simulink model "simulator_quarternions"  (R2025b)
settings: Solver=FixedStepAuto  StartTime=0.0  StopTime=15  FixedStep=0.01  RelTol=1e-3
values from neighbouring files (symbols this model uses):
  omega0 = qdot0    [model_init.m]
  q0_quat = euler2quat(q0)    [model_init.m]
  u0 = system_params.u0(i)    [Q_tension_calc.m]    (also in Tau_tension_calc.m; model_init.m = u0_calc(q0, system_params); u0_calc.m = zeros(size(fields)))
  u_offset = [106; 80; 79; 75; 67; 72; 80]/1000 - u0_calc(q_neutral, system_params)    [model_init.m]
undefined symbols (not defined in the file or in its folder): Cd, Dd, EKF_settings, Jm, Ke, Km, Mf, Ml, P0, Ra, system_params, u0_mpc, x0_EKF
libraries: mpclib x1
settings Model: Creator=Sigbjørn  LastModifiedBy=sig

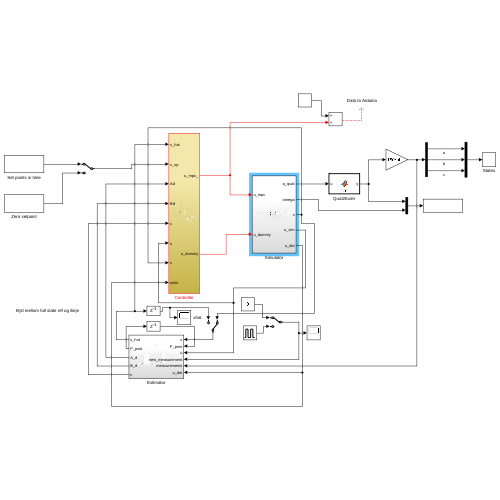
[thumbnail: Simulink's stored preview of the top-level diagram]
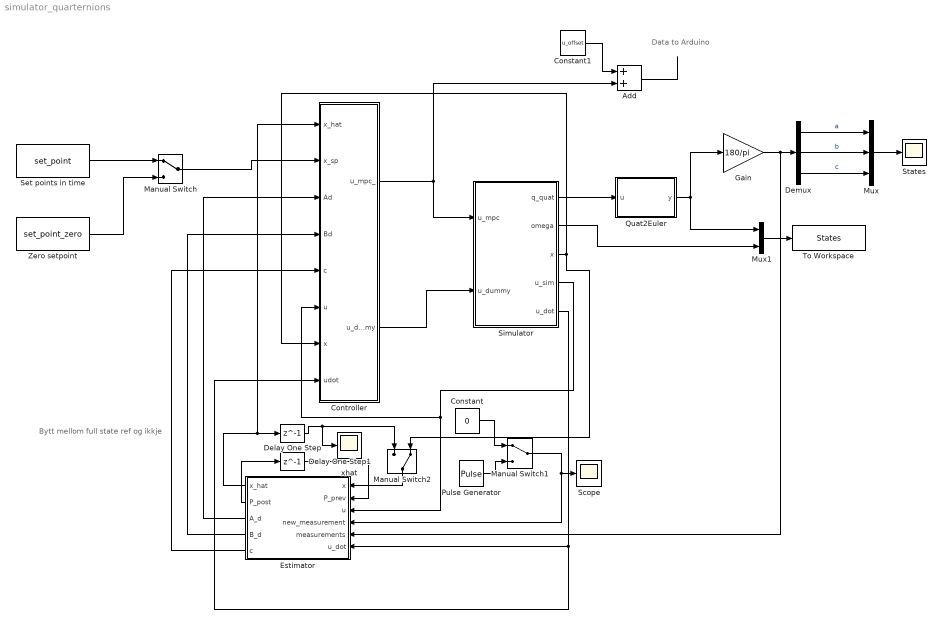
== system simulator_quarternions ==
  note: Bytt mellom full state ref og ikkje
  note: Data to Arduino
  Add : Sum
  Constant : Constant  Value=0
  Constant1 : Constant  Value=u_offset
  Controller : Subsystem
  Delay One Step : Delay  DelayLength=1  InitialCondition=x0_EKF
  Delay One Step1 : Delay  DelayLength=1  InitialCondition=P0
  Demux : Demux  Outputs=3
  Estimator : Subsystem
      settings: PortSchema="{\"entries\":[{\"content\":{\"sides\":[{\"content\":{\"connectorIds\":[\"Out1\",\"Out2\",\"Out3\",\"Out4\",\"Out5\"]},\"type\":\"ConnectorPlacement.EquallySpacedRectSide\",\"uuid\":\"f477ef40-4352-4d84-a45f-d7b8149414e1\"},{\"content\":{\"connectorIds\":[\"In1\",\"In2\",\"In3\",\"In4\",\"In5\",\"In6\"],\"side\":\"RIGHT\"},\"type\":\"ConnectorPlacement.EquallySpacedRectSide\",\"uuid\":\"8f29c47b-7819-47b7-a7db-3d460012710f\"},{\"content\":{\"side\":\"TOP\"},\"type\":\"ConnectorPlacement.EquallySpacedRectSide\",\"uuid\":\"6fcef62b-5cfa-49ba-93f4-5d540223ca0d\"}]},\"type\":\"ConnectorPlacement.EquallySpacedConnector\",\"uuid\":\"aa31ebfc-db05-4e23-be25-e9e271d34221\"}],\"packageUris\":[\"http://schema.mathworks.com/mf0/Connector/R2020b\"],\"version\":\"1.0\"}"
  Gain : Gain  Gain=180/pi
  Manual Switch : ManualSwitch
  Manual Switch1 : ManualSwitch
  Manual Switch2 : ManualSwitch  CurrentSetting=0
  Mux : Mux  Inputs=3
  Mux1 : Mux  Inputs=2
  Pulse Generator : DiscretePulseGenerator  PulseType=Time based  Period=0.02  PulseWidth=50
  Quat2Euler : MATLAB Function  TreatAsAtomicUnit=on
  Scope : Scope
      settings: ActiveDisplayYMinimum=-0.12120060790273554  ActiveDisplayYMaximum=1.1287993920972645  DataLoggingVariableName=ScopeData11
  Set points in time : FromWorkspace  VariableName=set_point
  Simulator : Subsystem
  States : Scope
      settings: ActiveDisplayYMinimum=-10.10714831247482  ActiveDisplayYMaximum=66.129260199609718
  To Workspace : ToWorkspace  VariableName=States  SaveFormat=Timeseries  SampleTime=-1
  Zero setpoint : FromWorkspace  VariableName=set_point_zero
  xhat : Scope
      settings: ActiveDisplayYMinimum=-1.0125974591295661  ActiveDisplayYMaximum=1.223621939903285  DataLoggingVariableName=ScopeData13
  wires:
  Demux/1 -> Mux/1  "a"
  Demux/2 -> Mux/2  "b"
  Demux/3 -> Mux/3  "c"
  Gain/1 -> Estimator/5(measurements), Demux/1
  Mux/1 -> States/1
  Manual Switch1/1 -> Estimator/4(new_measurement), Scope/1
  Estimator/2(P_post) -> Delay One Step1/1
  Delay One Step/1 -> Manual Switch2/1, xhat/1
  Delay One Step1/1 -> Estimator/2(P_prev)
  Estimator/3(A_d) -> Controller/3(Ad)
  Estimator/4(B_d) -> Controller/4(Bd)
  Estimator/1(x_hat) -> Controller/1(x_hat), Delay One Step/1
  Estimator/5(c) -> Controller/5(c)
  Set points in time/1 -> Manual Switch/1
  Controller/2(u_dummy) -> Simulator/2(u_dummy)
  Quat2Euler/1(y) -> Gain/1, Mux1/1
  Simulator/1(q_quat) -> Quat2Euler/1(u)
  Manual Switch/1 -> Controller/2(x_sp)
  Zero setpoint/1 -> Manual Switch/2
  Simulator/2(omega) -> Mux1/2
  Mux1/1 -> To Workspace/1
  Simulator/3(x) -> Manual Switch2/2, Controller/7(x)
  Pulse Generator/1 -> Manual Switch1/2
  Constant/1 -> Manual Switch1/1
  Constant1/1 -> Add/1
  Add/1 -> ?
  Controller/1(u_mpc_) -> Add/2, Simulator/1(u_mpc)
  Simulator/4(u_sim) -> Estimator/3(u), Controller/6(u)
  Manual Switch2/1 -> Estimator/1(x)
  Simulator/5(u_dot) -> Controller/8(udot), Estimator/6(u_dot)

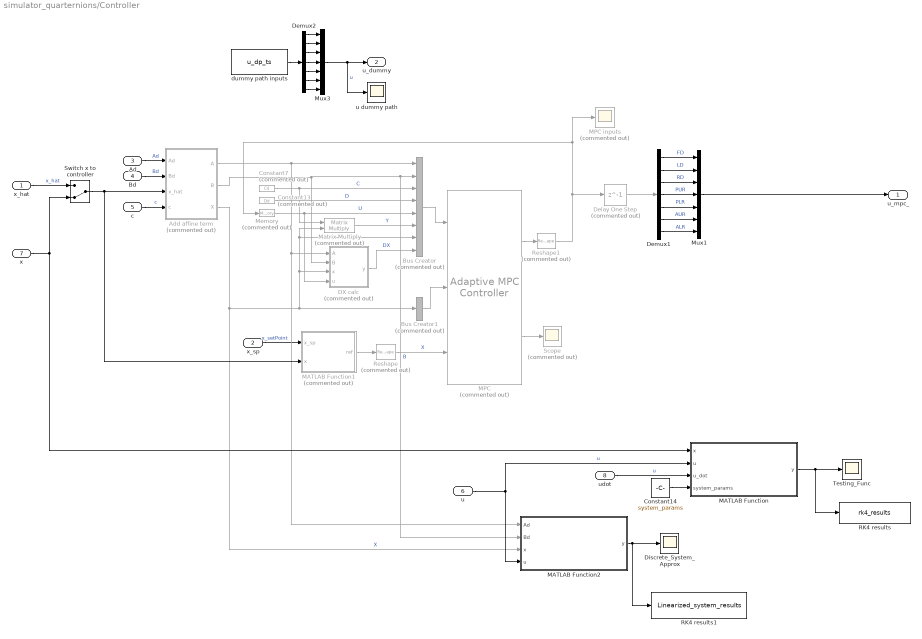
== system simulator_quarternions/Controller ==
  x_hat : Inport
  x_sp : Inport  Port=2
  Ad : Inport  Port=3
  Bd : Inport  Port=4
  c : Inport  Port=5
  u : Inport  Port=6
  x : Inport  Port=7
  udot : Inport  Port=8
  Add affine term : MATLAB Function  Commented=on  TreatAsAtomicUnit=on
  Bus Creator : BusCreator  Commented=on  Inputs=8
  Bus Creator1 : BusCreator  Commented=on  Inputs=1
  Constant13 : Constant  Commented=on  Value=Dd
  Constant14 : Constant  Value=system_params  OutDataTypeStr=Bus: System_params_bus
  Constant7 : Constant  Commented=on  Value=Cd
  DX calc : MATLAB Function  Commented=on  TreatAsAtomicUnit=on
  Delay One Step : Delay  Commented=on  DelayLength=1  InitialCondition=u0_mpc
  Demux1 : Demux  Outputs=7
  Demux2 : Demux  Outputs=7
  Discrete_System_Approx : Scope
      settings: ActiveDisplayYMinimum=-402.00121405870453  ActiveDisplayYMaximum=118.02698100135055  DataLoggingVariableName=ScopeData18
  MATLAB Function : MATLAB Function  TreatAsAtomicUnit=on
  MATLAB Function1 : MATLAB Function  Commented=on  TreatAsAtomicUnit=on
  MATLAB Function2 : MATLAB Function  TreatAsAtomicUnit=on
  MPC : mpclib/Adaptive MPC Controller  Commented=on  SCDEnableBlockLinearizationSpecification=on  mpcobj=MPC_controller  enable_value=0  updateMPCinCallerWorkspace=on  md_inport=off  mv_inport=off  uref_inport=off  return_cost=on  return_mvseq=off  return_qpstatus=off  return_xseq=off  return_state=off  return_ovseq=off  state_inport=on  isltv_plant=off  umin_inport=off  umax_inport=off  ymin_inport=off  ymax_inport=off  cc_inport=off  ywt_inport=off  uwt_inport=off  duwt_inport=off  rhoeps_inport=off  pm_inport=off  MaximumP=10  HorizonChoice=FixedHorizon  BlockDataType=double  SampleTimeInherited=off  switch_inport=off
  MPC inputs : Scope  Commented=on
      settings: ActiveDisplayYMinimum=-0.12500000000364678  ActiveDisplayYMaximum=1.1250000000004621
  Matrix Multiply : Product  Commented=on  Multiplication=Matrix(*)
  Memory : Memory  Commented=on  InitialCondition=u0_mpc
  Mux1 : Mux  Inputs=7
  Mux3 : Mux  Inputs=7
  RK4 results : ToWorkspace  VariableName=rk4_results  SaveFormat=Timeseries  SampleTime=-1
  RK4 results1 : ToWorkspace  VariableName=Linearized_system_results  SaveFormat=Timeseries  SampleTime=-1
  Reshape : Reshape  Commented=on  OutputDimensionality=Column vector (2-D)
  Reshape1 : Reshape  Commented=on  OutputDimensionality=Column vector (2-D)
  Scope : Scope  Commented=on
      settings: ActiveDisplayYMinimum=-3.0915324853365227E+10  ActiveDisplayYMaximum=2.7823792368028711E+11  DataLoggingVariableName=ScopeData19
  Switch x to controller : ManualSwitch  CurrentSetting=0
  Testing_Func : Scope
      settings: ActiveDisplayYMinimum=-0.58112707669885177  ActiveDisplayYMaximum=1.1756807862998724  DataLoggingVariableName=ScopeData16
  dummy path inputs : FromWorkspace  VariableName=u_dp_ts
  u dummy path : Scope
      settings: ActiveDisplayYMinimum=0.093690576639966744  ActiveDisplayYMaximum=0.20938778318519038  DataLoggingVariableName=ScopeData24
  u_mpc_ : Outport
  u_dummy : Outport  Port=2
  wires:
  Ad/1 -> Add affine term/1(Ad)  "Ad"
  Add affine term/2(B) -> MATLAB Function2/2(Bd), Bus Creator/2, DX calc/2(B)  "B"
  x_sp/1 -> MATLAB Function1/1(x_sp)  "x_setPoint"
  MPC/1 -> Reshape1/1
  Bus Creator/1 -> MPC/1
  Bus Creator1/1 -> MPC/2
  Constant7/1 -> Bus Creator/3, Matrix Multiply/1  "C"
  Constant13/1 -> Bus Creator/4  "D"
  Matrix Multiply/1 -> Bus Creator/6  "Y"
  DX calc/1(y) -> Bus Creator/8  "DX"
  Reshape1/1 -> MPC inputs/1, Memory/1, Delay One Step/1
  Demux1/7 -> Mux1/7  "ALR"
  Demux1/6 -> Mux1/6  "AUR"
  Demux1/5 -> Mux1/5  "PLR"
  Demux1/4 -> Mux1/4  "PUR"
  Demux1/3 -> Mux1/3  "RD"
  Demux1/2 -> Mux1/2  "LD"
  Demux1/1 -> Mux1/1  "FD"
  MATLAB Function/1(y) -> RK4 results/1, Testing_Func/1
  Constant14/1 -> MATLAB Function/4(system_params)
  c/1 -> Add affine term/4(c)  "c"
  Add affine term/3(X) -> MATLAB Function2/3(x), Bus Creator1/1, DX calc/3(x), Bus Creator/7, Matrix Multiply/2  "X"
  Memory/1 -> DX calc/4(u), Bus Creator/5  "U"
  Reshape/1 -> MPC/3  "X"
  Add affine term/1(A) -> MATLAB Function2/1(Ad), DX calc/1(A), Bus Creator/1
  Bd/1 -> Add affine term/2(Bd)  "Bd"
  x_hat/1 -> Switch x to controller/1  "x_hat"
  Mux1/1 -> u_mpc_/1
  Delay One Step/1 -> Demux1/1
  Switch x to controller/1 -> MATLAB Function1/2(x), Add affine term/3(x_hat)
  u/1 -> MATLAB Function2/4(u), MATLAB Function/2(u)  "u"
  x/1 -> Switch x to controller/2, MATLAB Function/1(x)
  MPC/2 -> Scope/1
  dummy path inputs/1 -> Demux2/1
  Mux3/1 -> u_dummy/1, u dummy path/1  "u"
  Demux2/3 -> Mux3/3
  Demux2/5 -> Mux3/5
  Demux2/7 -> Mux3/7
  Demux2/2 -> Mux3/2
  Demux2/6 -> Mux3/6
  Demux2/4 -> Mux3/4
  Demux2/1 -> Mux3/1
  MATLAB Function2/1(y) -> RK4 results1/1, Discrete_System_Approx/1
  MATLAB Function1/1(ref) -> Reshape/1
  udot/1 -> MATLAB Function/3(u_dot)  "u"

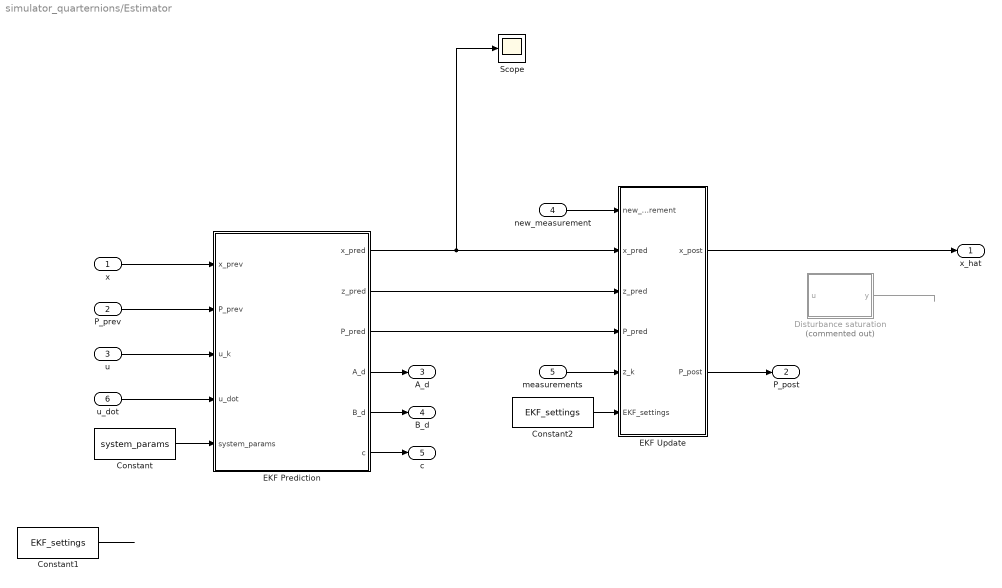
== system simulator_quarternions/Estimator ==
  x : Inport
  P_prev : Inport  Port=2
  u : Inport  Port=3
  new_measurement : Inport  Port=4
  measurements : Inport  Port=5
  u_dot : Inport  Port=6
  Constant : Constant  Value=system_params  OutDataTypeStr=Bus: System_params_bus
  Constant1 : Constant  Value=EKF_settings  OutDataTypeStr=Bus: EKFBus
  Constant2 : Constant  Value=EKF_settings  OutDataTypeStr=Bus: EKFBus
  Disturbance saturation : MATLAB Function  Commented=on  TreatAsAtomicUnit=on
  EKF Prediction : MATLAB Function  TreatAsAtomicUnit=on
  EKF Update : MATLAB Function  TreatAsAtomicUnit=on
  Scope : Scope
      settings: ActiveDisplayYMinimum=-1  ActiveDisplayYMaximum=1  DataLoggingVariableName=ScopeData12
  x_hat : Outport
  P_post : Outport  Port=2
  A_d : Outport  Port=3
  B_d : Outport  Port=4
  c : Outport  Port=5
  wires:
  x/1 -> EKF Prediction/1(x_prev)
  EKF Update/1(x_post) -> x_hat/1
  u/1 -> EKF Prediction/3(u_k)
  P_prev/1 -> EKF Prediction/2(P_prev)
  Constant/1 -> EKF Prediction/5(system_params)
  EKF Prediction/1(x_pred) -> Scope/1, EKF Update/2(x_pred)
  EKF Prediction/2(z_pred) -> EKF Update/3(z_pred)
  EKF Prediction/3(P_pred) -> EKF Update/4(P_pred)
  EKF Prediction/4(A_d) -> A_d/1
  EKF Prediction/5(B_d) -> B_d/1
  new_measurement/1 -> EKF Update/1(new_measurement)
  EKF Update/2(P_post) -> P_post/1
  measurements/1 -> EKF Update/5(z_k)
  EKF Prediction/6(c) -> c/1
  Constant1/1 -> ?
  Constant2/1 -> EKF Update/6(EKF_settings)
  Disturbance saturation/1(y) -> ?
  u_dot/1 -> EKF Prediction/4(u_dot)

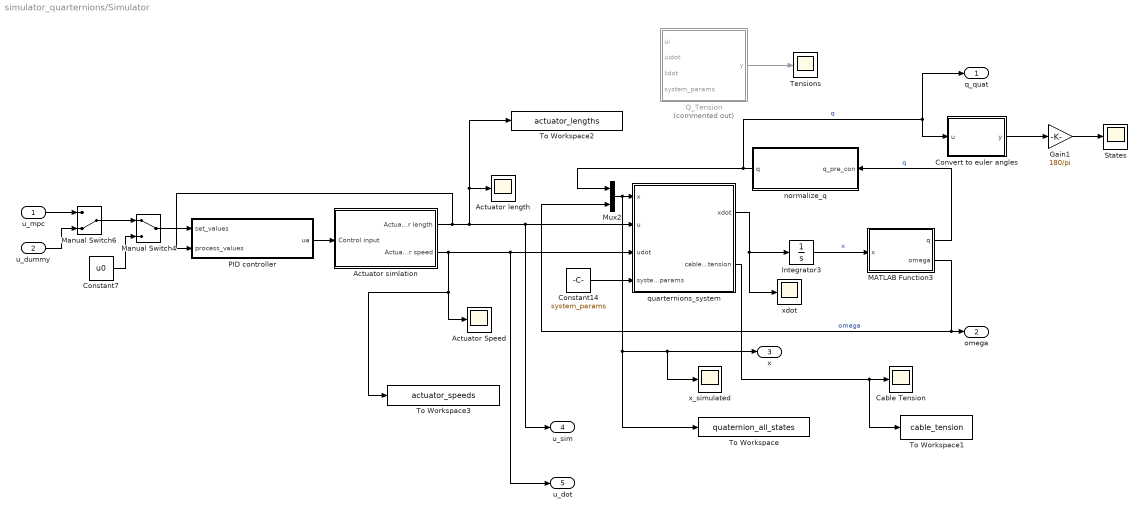
== system simulator_quarternions/Simulator ==
  u_mpc : Inport
  u_dummy : Inport  Port=2
  Actuator Speed : Scope
      settings: ActiveDisplayYMinimum=-0.0014664190047903012  ActiveDisplayYMaximum=0.013197771043112715  DataLoggingVariableName=ScopeData7
  Actuator length : Scope
      settings: ActiveDisplayYMinimum=0.11825035541108625  ActiveDisplayYMaximum=0.27502608509431004  DataLoggingVariableName=ScopeData3
  Actuator simlation : Subsystem
  Cable Tension : Scope
      settings: ActiveDisplayYMinimum=-1  ActiveDisplayYMaximum=1  DataLoggingVariableName=ScopeData8
  Constant14 : Constant  Value=system_params  OutDataTypeStr=Bus: System_params_bus
  Constant7 : Constant  Value=u0
  Convert to euler angles : MATLAB Function  TreatAsAtomicUnit=on
  Gain1 : Gain  Gain=180/pi
  Integrator3 : Integrator  InitialCondition=[q0_quat;omega0]
  MATLAB Function3 : MATLAB Function  TreatAsAtomicUnit=on
  Manual Switch4 : ManualSwitch
  Manual Switch6 : ManualSwitch  CurrentSetting=0
  Mux2 : Mux  Inputs=2
  PID controller : MATLAB Function  TreatAsAtomicUnit=on
  Q_Tension : MATLAB Function  Commented=on  TreatAsAtomicUnit=on
  States : Scope
      settings: ActiveDisplayYMinimum=-43.174853082907831  ActiveDisplayYMaximum=84.845575307980468  DataLoggingVariableName=ScopeData27
  Tensions : Scope
      settings: DataLoggingVariableName=ScopeData23
  To Workspace : ToWorkspace  VariableName=quaternion_all_states  SaveFormat=Timeseries  SampleTime=-1
  To Workspace1 : ToWorkspace  VariableName=cable_tension  SaveFormat=Timeseries  SampleTime=-1
  To Workspace2 : ToWorkspace  VariableName=actuator_lengths  SaveFormat=Timeseries  SampleTime=-1
  To Workspace3 : ToWorkspace  VariableName=actuator_speeds  SaveFormat=Timeseries  SampleTime=-1
  normalize_q : MATLAB Function  TreatAsAtomicUnit=on
  quarternions_system : MATLAB Function  TreatAsAtomicUnit=on
  x_simulated : Scope
      settings: ActiveDisplayYMinimum=-0.12499999999999997  ActiveDisplayYMaximum=1.125  DataLoggingVariableName=ScopeData2
  xdot : Scope
      settings: ActiveDisplayYMinimum=-15.47778972600711  ActiveDisplayYMaximum=15.477652119582009  DataLoggingVariableName=ScopeData28
  q_quat : Outport
  omega : Outport  Port=2
  x : Outport  Port=3
  u_sim : Outport  Port=4
  u_dot : Outport  Port=5
  wires:
  Constant14/1 -> quarternions_system/4(system_params)
  u_mpc/1 -> Manual Switch6/1
  Constant7/1 -> Manual Switch4/2
  Q_Tension/1(y) -> Tensions/1
  u_dummy/1 -> Manual Switch6/2
  Manual Switch6/1 -> Manual Switch4/1
  quarternions_system/1(xdot) -> xdot/1, Integrator3/1
  Integrator3/1 -> MATLAB Function3/1(x)  "x"
  MATLAB Function3/1(q) -> normalize_q/1(q_pre_con)  "q"
  normalize_q/1(q) -> Mux2/1, Convert to euler angles/1(u), q_quat/1  "q"
  MATLAB Function3/2(omega) -> omega/1, Mux2/2  "omega"
  Mux2/1 -> To Workspace/1, x_simulated/1, x/1, quarternions_system/1(x)
  Gain1/1 -> States/1
  Convert to euler angles/1(y) -> Gain1/1
  PID controller/1(ua) -> Actuator simlation/1(Control input)
  Manual Switch4/1 -> PID controller/1(set_values)
  Actuator simlation/1(Actuator length) -> To Workspace2/1, Actuator length/1, u_sim/1, quarternions_system/2(u), PID controller/2(process_values)
  Actuator simlation/2(Actuator speed) -> u_dot/1, quarternions_system/3(udot), Actuator Speed/1, To Workspace3/1
  quarternions_system/2(cable_tension) -> To Workspace1/1, Cable Tension/1

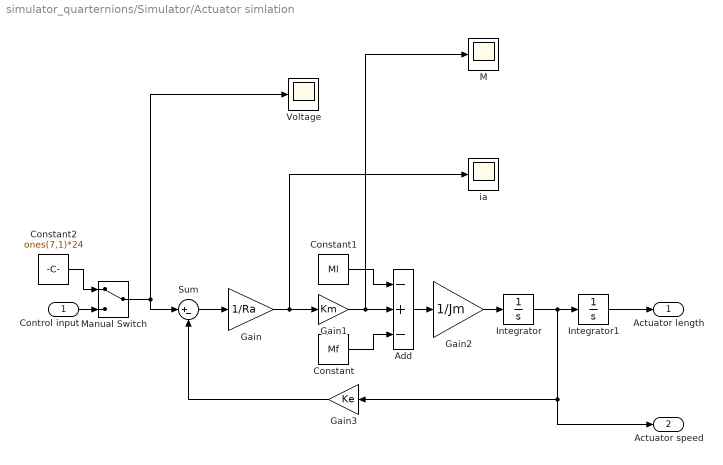
== system simulator_quarternions/Simulator/Actuator simlation ==
  Control input : Inport
  Add : Sum  Inputs=-+-
  Constant : Constant  Value=Mf
  Constant1 : Constant  Value=Ml
  Constant2 : Constant  Value=ones(7,1)*24
  Gain : Gain  Gain=1/Ra
  Gain1 : Gain  Gain=Km
  Gain2 : Gain  Gain=1/Jm
  Gain3 : Gain  Gain=Ke
  Integrator : Integrator  InitialCondition=zeros(7,1)
  Integrator1 : Integrator  InitialCondition=u0
  M : Scope
      settings: ActiveDisplayYMinimum=-4.2156377432993638E+304  ActiveDisplayYMaximum=4.6840958424388109E+303  DataLoggingVariableName=ScopeData5
  Manual Switch : ManualSwitch
  Sum : Sum  Inputs=|+-
  Voltage : Scope
      settings: ActiveDisplayYMinimum=-30  ActiveDisplayYMaximum=30  DataLoggingVariableName=ScopeData4
  ia : Scope
      settings: ActiveDisplayYMinimum=-2.9766820323850531E+30  ActiveDisplayYMaximum=3.3074625433172575E+29  DataLoggingVariableName=ScopeData6
  Actuator length : Outport
  Actuator speed : Outport  Port=2
  wires:
  Manual Switch/1 -> Voltage/1, Sum/1
  Integrator1/1 -> Actuator length/1
  Integrator/1 -> Actuator speed/1, Gain3/1, Integrator1/1
  Gain2/1 -> Integrator/1
  Add/1 -> Gain2/1
  Gain1/1 -> M/1, Add/2
  Gain/1 -> ia/1, Gain1/1
  Sum/1 -> Gain/1
  Gain3/1 -> Sum/2
  Constant/1 -> Add/3
  Constant1/1 -> Add/1
  Control input/1 -> Manual Switch/2
  Constant2/1 -> Manual Switch/1

== matlab function simulator_quarternions/Estimator/Disturbance saturation ==
  data: u input; y output
function y = fcn(u)
lLim = -0.1;
uLim = 0.1;

for i=7:9
    if u(i) > uLim
        u(i) = uLim;
    elseif u(i) < lLim
        u(i) = lLim;
    end
end
y = u;

== matlab function simulator_quarternions/Simulator/Q_Tension ==
  data: ui input; y output; uidot input; lidot input; system_params input
function y = fcn(ui, uidot, lidot, system_params)
R_h = Rot_mat(q);
R_hxy = Rot_xy(q);
Q = zeros(3,1);
fields = fieldnames(system_params.cables);

for i = 1:numel(fields)
    cable = system_params.cables.(fields{i});
    %if i < 4
        ri = - R_h*cable.L + cable.M;
        %ri = R_h*cable.L - cable.M;
        rpli = R_h * cable.L;
        % Calc drdq
        drdq_ = drdq(q, rpli);
        
    % else
    %     ri = - R_hxy*cable.L + cable.M;
    %     ri = R_hxy*cable.L - cable.M;
    %     rpli = R_hxy * cable.L;
    %     % Calc drdq
    %     drdq_ = drdq(q, rpli);
    % 
    % end
    li = norm(ri);
    di = ri/li;
    dldq = zeros(3,1);
    for j = 1:3
        dldq(j) = di'*drdq_(:,j);
    end
    drdq_;
    lidot = dldq'*qdot;
    %lidot_check = dot(di, cross(omega, p_i));
    % numerical derivative
    eps = 1e-6;
    q_eps = q + qdot * eps;
    
    % recompute length at slightly forward time
    R_eps = Rot_mat(q_eps);
    r_eps = R_eps * cable.L -cable.M;
    l_eps = norm(r_eps);
    
    lidot_num = (l_eps - li)/eps;

    dldq_num = zeros(3,1);
    
    for j = 1:3
        dq = zeros(3,1);
        dq(j) = eps;
    
        q_eps = q + dq;
    
        % recompute rotation
        R_eps = Rot_mat(q_eps);
    
        % recompute cable vector (IMPORTANT: same definition as ri)
        %if i < 4
             ri_eps = R_eps * cable.L - cable.M;
        % else
        %     Rxy_eps = Rot_xy(q_eps);
        %     ri_eps = Rxy_eps * cable.L - cable.M;
        % end
    
        li_eps = norm(ri_eps);
    
        dldq_num(j) = (li_eps - li) / eps;
    end
    
    % Compare
    lidot;
    lidot_num;
    %disp('Analytical vs Numerical dldq:')
    %disp([dldq, dldq_num])
    
    dldq;
    di;
    drdq_;
    T = Tension(u(i), li, udot(i), lidot, system_params);
    
y = Tension(ui, li, uidot, lidot, system_params);

== matlab function simulator_quarternions/Simulator/quarternions_system ==
  data: x input; u input; udot input; xdot output; system_params input; cable_tension output
function [xdot, cable_tension] = fcn(x, u, udot, system_params)
xdot = system_model_quat_omega(x, u, udot, system_params);

% Tension calculation
q = x(1:4);
omega = x(5:7);
R = quat2rotm(q);
R_humerus = system_params.Rhum;

fields = fieldnames(system_params.cables);

cable_tension = zeros(7,1);

for i = 1:numel(fields)
    cable = system_params.cables.(fields{i});
    p_humerus = R * cable.L;
    p_scapula = cable.M;

    ri = p_humerus;
    di = p_scapula - ri;
        
    li = norm(di);
    di_hat = di/li;

    % Check for cable-humerus collision
    n = di'*p_humerus;
    d = di'*di;
    t_star = -n/d;
    p_closest = p_humerus + t_star * di;
    p_norm = norm(p_closest);
    p_hat = p_closest/p_norm;
    
    if p_norm < R_humerus
    
   
        % Create wrapping point
        p_wrap = p_closest/p_norm * R_humerus;
        v = cable.v;

        if dot(p_wrap, v) < -1e-6
            p_wrap = p_wrap - 2 * dot(p_wrap, v) * v;
        end

        li = norm(p_humerus - p_wrap) + norm(p_scapula - p_wrap);

        p_humerus_dot = cross(omega, p_humerus);
        di_dot = -p_humerus_dot;
        n_dot = di_dot'*p_humerus + di'*p_humerus_dot;
        d_dot = 2*di'*di_dot;
        t_star_dot = -n_dot/d + n/d^2 * d_dot;
        p_closest_dot = p_humerus_dot + t_star_dot*di + t_star*di_dot;
        p_wrap_dot = R_humerus/p_norm * (eye(3)-p_hat*p_hat')*p_closest_dot;
        term1 = (p_humerus-p_wrap)'/norm(p_humerus-p_wrap)*(p_humerus_dot-p_wrap_dot);
        term2 = (p_scapula-p_wrap)'/norm(p_scapula-p_wrap)*-p_wrap_dot;
        lidot = term1 + term2; 

        di = p_wrap - p_humerus;
        di_hat = di/norm(di);
    else
        % Calculate as normal
        lidot = -di_hat' * cross(omega, ri);
    end
        
    
    u0 = system_params.u0(i);

    cable_tension(i) = Tension(u(i), u0, li, udot(i), lidot, system_params);
end

== matlab function simulator_quarternions/Simulator/MATLAB Function3 ==
  data: x input; q output; omega output
function [q, omega] = fcn(x)
q = x(1:4);
omega = x(5:7);

== matlab function simulator_quarternions/Simulator/normalize_q ==
  data: q_pre_con input; q output
function q = fcn(q_pre_con)
q = q_pre_con/norm(q_pre_con);

== matlab function simulator_quarternions/Simulator/Convert to euler angles ==
  data: u input; y output
function y = fcn(u)
y = quat2euler(u);

== matlab function simulator_quarternions/Quat2Euler ==
  data: u input; y output
function y = fcn(u)
y = quat2euler(u);

== matlab function simulator_quarternions/Controller/MATLAB Function1 ==
  data: x_sp input; ref output; x input
function ref = fcn(x_sp, x)

q = x(1:4);
q_sp = x_sp(1:4);

if dot(q, q_sp) < 0
    q_ref = -q_sp;
else
    q_ref = q_sp;
end

ref = [q_ref; x(5:7)];

== matlab function simulator_quarternions/Simulator/PID controller ==
  data: set_values input; ua output; process_values input
function ua = fcn(set_values, process_values)
% Pure P controller
kp = ones(7,1)*4;

errors = set_values - process_values;
errors = errors * 1000; % Convert to mm

controller_bias = 64;
u_controller = errors.*kp + controller_bias;

% Saturate
for i = 1:7
    if u_controller(i) < 0
        u_controller(i) = 0;
    elseif u_controller(i) > 127
        u_controller(i) = 127;
    end
end

% Transform to voltage
ua = (24 + 24)/127 * u_controller - 24;

== matlab function simulator_quarternions/Estimator/EKF Prediction ==
  data: x_prev input; x_pred output; P_prev input; u_k input; u_dot input; z_pred output; P_pred output; A_d output; B_d output; system_params input; c output; EKF_settings parameter
function [x_pred, z_pred, P_pred, A_d, B_d, c] = fcn(x_prev, P_prev, u_k, u_dot, system_params, EKF_settings)

%[x_pred, z_pred, P_pred, A_d, B_d, c] = EKF_pred(x_prev, P_prev, u_k, u_dot, EKF_settings, system_params);
[x_pred, z_pred, P_pred, A_d, B_d, c] = EKF_pred_quaternions(x_prev, P_prev, u_k, u_dot, EKF_settings, system_params);

== matlab function simulator_quarternions/Estimator/EKF Update ==
  data: new_measurement input; x_pred input; z_pred input; x_post output; P_pred input; z_k input; EKF_settings input; P_post output
function [x_post,P_post] = fcn(new_measurement, x_pred, z_pred, P_pred, z_k, EKF_settings)
persistent isInitialized
if isempty(isInitialized)
    x_pred = EKF_settings.x0;
    P_pred = EKF_settings.P0;
    isInitialized = true;
end

if new_measurement
    %[x_post,P_post] = EKF_upd(x_pred, P_pred, z_pred, z_k, EKF_settings);
    [x_post,P_post] = EKF_upd_quaternions(x_pred, P_pred, z_pred, z_k, EKF_settings);
else
    x_post = x_pred;
    P_post = P_pred;
end

== matlab function simulator_quarternions/Controller/DX calc ==
  data: A input; B input; x input; u input; y output
function y = fcn(A,B,x,u)
y = A*x + B*u - x;

== matlab function simulator_quarternions/Controller/MATLAB Function ==
  data: x input; u input; u_dot input; y output; system_params input
function y = fcn(x,u, u_dot,system_params)
%y = system_model_continous(x, u, system_params);
y = runge_kutta4(x, u, u_dot, 0.01, system_params);

== matlab function simulator_quarternions/Controller/MATLAB Function2 ==
  data: Ad input; Bd input; x input; u input; y output
function y = fcn(Ad,Bd,x,u)
y = Ad*x + Bd*u;
%y = Ad*x;
%disp(Ad)
%disp(Bd)

== matlab function simulator_quarternions/Controller/Add affine term ==
  data: Ad input double; A output; Bd input; x_hat input; B output; X output; c input
function [A,B,X] = fcn(Ad,Bd,x_hat,c)
A = [Ad c; zeros(1,size(Ad,1)) 0];
B = [Bd; zeros(1,size(Bd,2))];
X = [x_hat;1];
